simulink model "identificacao"  (R2018b)
settings: Solver=ode4  StartTime=0.0  StopTime=100  FixedStep=0.002  RelTol=1e-3  EnableMultiTasking=on
libraries: arduinolib x4, simulink x4
settings Model: ExtModeTrigDuration=2  Creator=pedro  LastModifiedBy=pedro
settings SolverCC: AutoInsertRateTranBlk=on
settings OptimizationCC: EnhancedBackFolding=on  PassReuseOutputArgsAs=Individual arguments  MaxStackSize=64  OptimizeBlockOrder=speed  DifferentSizesBufferReuse=on  OptimizationCustomize=off
settings DebuggingCC: ParameterTunabilityLossMsg=error
settings HardwareCC: ProdBitPerInt=16  ProdBitPerPointer=16  ProdBitPerSizeT=16  ProdBitPerPtrDiffT=16  ProdLargestAtomicFloat=None  ProdWordSize=8  ProdHWDeviceType=Atmel->AVR  UseEmbeddedCoderFeatures=off  UseSimulinkCoderFeatures=off
settings SFSimCC: SimUseLocalCustomCode=off  MATLABDynamicMemAlloc=off
settings RTWCC: SystemTargetFile=ert.tlc  HardwareBoard=Arduino Mega 2560  TemplateMakefile=ert_default_tmf  GenerateReport=on  RTWUseLocalCustomCode=off  Toolchain=Arduino AVR  BuildConfiguration=Faster Runs  IncludeHyperlinkInReport=on  LaunchReport=on  GenerateTraceInfo=on  GenerateTraceReport=on  GenerateTraceReportSl=on  GenerateTraceReportSf=on  GenerateTraceReportEml=on
settings CodeAppCC: ForceParamTrailComments=on  IgnoreCustomStorageClasses=off  OperatorAnnotations=on  SimulinkDataObjDesc=on  SFDataObjDesc=on  InsertBlockDesc=on
settings ERTTargetCC: SupportContinuousTime=on  SupportNonInlinedSFcns=on  SupportVariableSizeSignals=on

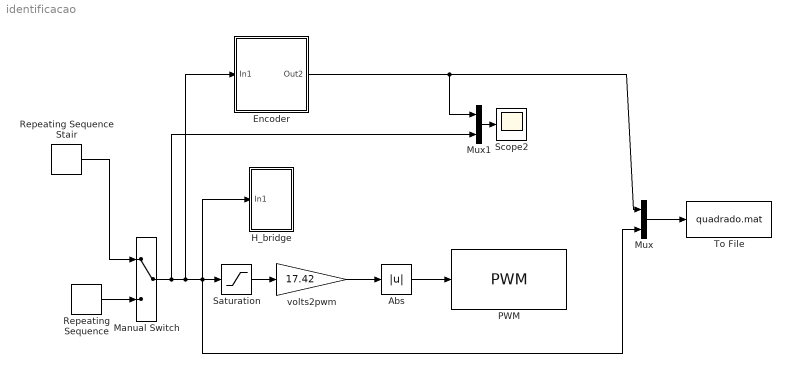
== system identificacao ==
  Abs : Abs
  Encoder : Subsystem
  "H_bridge " : Subsystem
  Manual Switch : ManualSwitch
  Mux : Mux  Inputs=2
  Mux1 : Mux  Inputs=2
  PWM : arduinolib/PWM  pinNumber=8  EnableInputFrequency=off  InitialFrequency=2000  InitialDutyCycle=0  NotificationType=None  blockPlatform=arduino
  Repeating Sequence : simulink/Sources/Repeating Sequence  rep_seq_t=[0 0.5 1 1.5 2]  rep_seq_y=[0 2 0 -2 0]
  Repeating Sequence Stair : simulink/Sources/Repeating Sequence Stair  OutValues=[2 -2]  tsamp=0.15  OutMin=[]  OutMax=[]  OutDataTypeStr=double  OutputDataTypeScalingMode=double  OutDataType=fixdt(0,8)  ConRadixGroup=Best Precision: Vector-wise  OutScaling=2^-12
  Saturation : Saturate  UpperLimit=14  LowerLimit=-14
  Scope2 : Scope
  To File : ToFile  Filename=quadrado.mat
  "volts2pwm " : Gain  Gain=17.42
  wires:
  Mux/1 -> To File/1
  Repeating Sequence/1 -> Manual Switch/2
  "volts2pwm "/1 -> Abs/1
  Saturation/1 -> "volts2pwm "/1
  Abs/1 -> PWM/1
  Manual Switch/1 -> Encoder/1(In1), Mux/2, "H_bridge "/1(In1), Saturation/1, Mux1/2
  Encoder/1(Out2) -> Mux/1, Mux1/1
  Mux1/1 -> Scope2/1
  Repeating Sequence Stair/1 -> Manual Switch/1

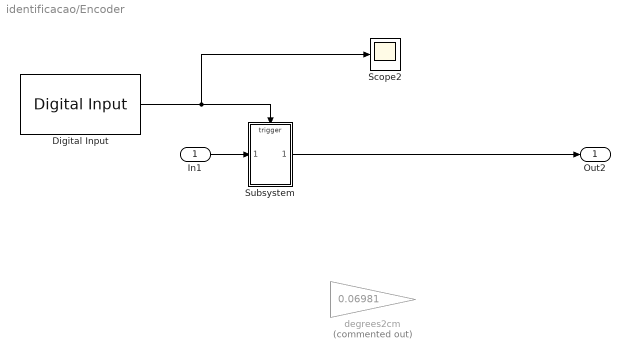
== system identificacao/Encoder ==
  In1 : Inport
  Digital Input : arduinolib/Digital Input  pinNumber=2  sampleTime=0.002  blockPlatform=arduino
      settings: SourceProductName=Simulink Support Package for Arduino Hardware
  Scope2 : Scope
  Subsystem : Subsystem
  degrees2cm : Gain  Commented=on  Gain=0.06981
  Out2 : Outport
  wires:
  In1/1 -> Subsystem/1(In1)
  Digital Input/1 -> Scope2/1, Subsystem/Trigger
  Subsystem/1(Out1) -> Out2/1

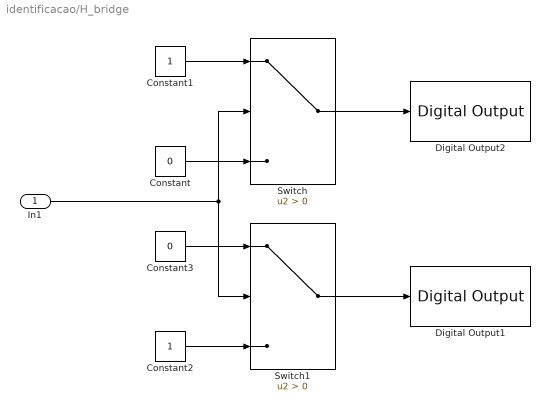
== system identificacao/H_bridge  ==
  In1 : Inport
  Constant : Constant  Value=0
  Constant1 : Constant
  Constant2 : Constant
  Constant3 : Constant  Value=0
  Digital Output1 : arduinolib/Digital Output  pinNumber=35  blockPlatform=arduino
  Digital Output2 : arduinolib/Digital Output  pinNumber=34  blockPlatform=arduino
  Switch : Switch  Criteria=u2 > Threshold
  Switch1 : Switch  Criteria=u2 > Threshold
  wires:
  Constant/1 -> Switch/3
  Switch1/1 -> Digital Output1/1
  Constant1/1 -> Switch/1
  Switch/1 -> Digital Output2/1
  Constant2/1 -> Switch1/3
  In1/1 -> Switch1/2, Switch/2
  Constant3/1 -> Switch1/1

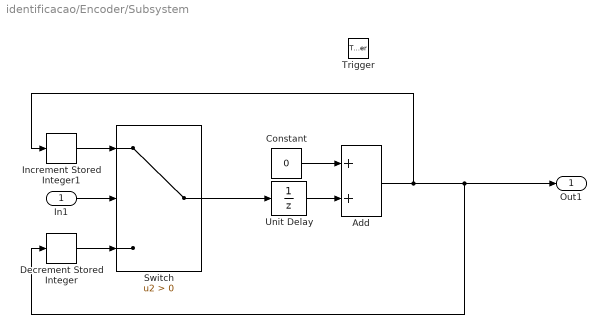
== system identificacao/Encoder/Subsystem ==
  In1 : Inport
  Trigger : TriggerPort  TriggerType=either  VariantControl=Variant  PortDimensions=1
  Add : Sum
  Constant : Constant  Value=0
  Decrement Stored Integer : simulink/Additional Math & Discrete/Additional Math: Increment - Decrement/Decrement Stored Integer
      settings: SourceProductName=Simulink  SourceProductBaseCode=SL
  Increment Stored Integer1 : simulink/Additional Math & Discrete/Additional Math: Increment - Decrement/Increment Stored Integer
      settings: SourceProductName=Simulink
  Switch : Switch  Criteria=u2 > Threshold
  Unit Delay : UnitDelay  SampleTime=-1
  Out1 : Outport
  wires:
  Add/1 -> Decrement Stored Integer/1, Out1/1, Increment Stored Integer1/1
  Constant/1 -> Add/1
  In1/1 -> Switch/2
  Decrement Stored Integer/1 -> Switch/3
  Increment Stored Integer1/1 -> Switch/1
  Switch/1 -> Unit Delay/1
  Unit Delay/1 -> Add/2
